simulink subsystem "PieroControladoPosicionz"  (R2023b)
settings: Solver=VariableStepAuto  StartTime=0.0  StopTime=10.0  RelTol=1e-3
undefined symbols (not defined in the file): DiscIntNeverNeededParam
settings Model: Creator=Antonio  LastModifiedBy=Antonio

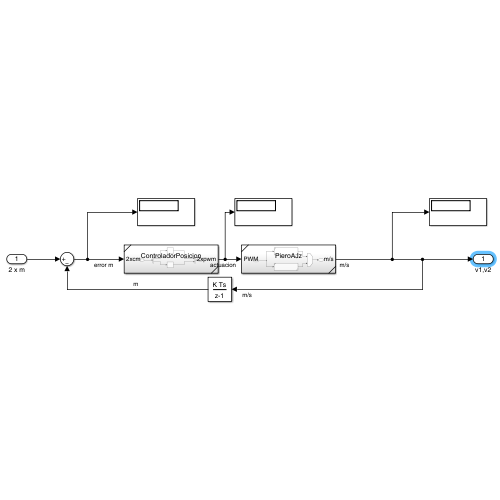
[thumbnail: Simulink's stored preview of the top-level diagram]
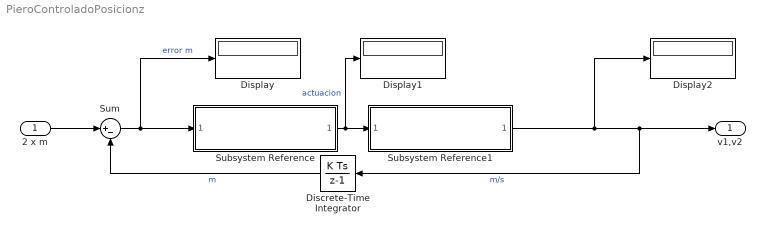
== system PieroControladoPosicionz ==
  2 x m : Inport
  Discrete-Time Integrator : DiscreteIntegrator  SampleTime=-1  ICPrevOutput=DiscIntNeverNeededParam  ICPrevScaledInput=DiscIntNeverNeededParam
  Display : Display
  Display1 : Display
  Display2 : Display
  Subsystem Reference : Subsystem  ReferencedSubsystem=ControladorPosicion
  Subsystem Reference1 : Subsystem  ReferencedSubsystem=PieroAJz
  Sum : Sum  Inputs=|+-
  v1,v2 : Outport
  wires:
  Discrete-Time Integrator/1 -> Sum/2  "m"
  Subsystem Reference1/1 -> Display2/1, Discrete-Time Integrator/1, v1,v2/1  "m/s"
  Sum/1 -> Display/1, Subsystem Reference/1  "error m"
  2 x m/1 -> Sum/1
  Subsystem Reference/1 -> Display1/1, Subsystem Reference1/1  "actuacion"
